simulink model "MIAC_Gain_or_disturbance_adaptive_test"  (R2018b)
settings: Solver=FixedStepDiscrete  StartTime=0.0  StopTime=60000  FixedStep=1  RelTol=1e-3
libraries: simulink x5, slident x5, powerlib_meascontrol x4
(part 2 of 3)

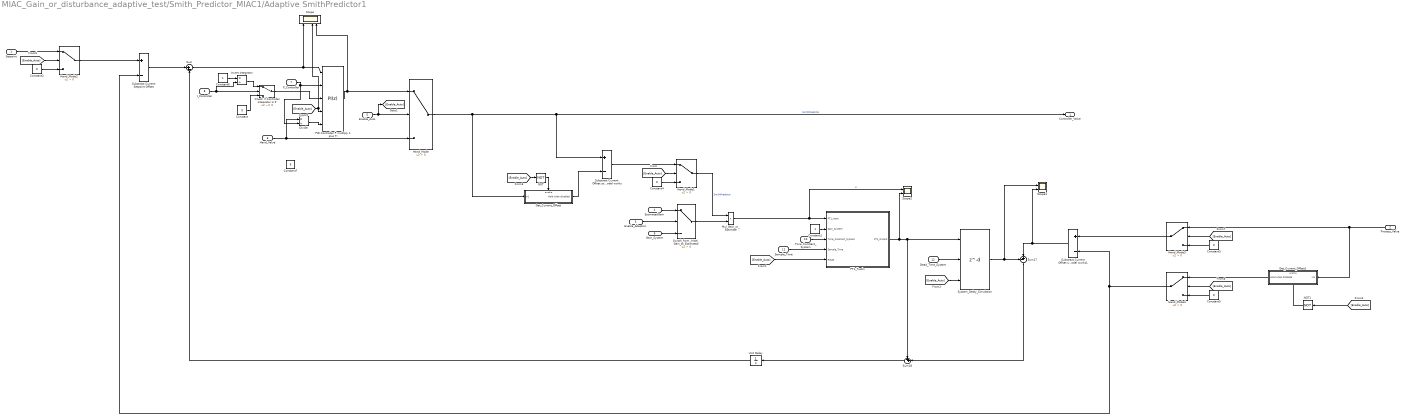
== system MIAC_Gain_or_disturbance_adaptive_test/Smith_Predictor_MIAC1/Adaptive SmithPredictor1 ==
  Setpoint : Inport
  Process_Value : Inport  Port=2
  Enable_Adaption : Inport  Port=3
  EstimatedGain : Inport  Port=4
  Enable_Auto : Inport  Port=5
  Hand_Value : Inport  Port=6
  P_Controller : Inport  Port=7
  I_Controller : Inport  Port=8
  Gain_System : Inport  Port=9
  Time_Constant_System : Inport  Port=10
  Sample_Time : Inport  Port=11
  " Dead_Time_System" : Inport  Port=12
  Check if Controller Integrator is 0 : Switch  Criteria=u2 ~= 0
  Constant{,2..5} (5 alike) : Constant  Value=0
  Constant1 : Constant
  Constant6 : Constant
  Constant7 : Constant  Value=6
  Divide : Product  Inputs=*/
  Get_Current_Offset : Subsystem
  Get_Current_Offset1 : Subsystem
  Hand_Mode{,1..4} (5 alike) : Switch  Criteria=u2 > Threshold
  Invert Integrator : Product  Inputs=*/
  Mul_Gain_or_Estimate : Product
  NOT : Logic  Operator=NOT  IconShape=distinctive  AllPortsSameDT=off  OutDataTypeStr=boolean
  NOT1 : Logic  Operator=NOT  IconShape=distinctive  AllPortsSameDT=off  OutDataTypeStr=boolean
  "PID Controller P multiply 1 plus Ti " : simulink/Continuous/PID Controller  Controller=PI  Form=Ideal  TimeDomain=Discrete-time  SampleTime=1  IntegratorMethod=Forward Euler  FilterMethod=Forward Euler  ControllerParametersSource=external  P=1.66148812255363  I=0.0833845225035065  D=118.272348286844  UseFilter=on  N=0.00420306193364532  TunerSelectOption=Transfer Function Based (PID Tuner App)  InitialConditionSource=external  InitialConditionForIntegrator=0  InitialConditionForFilter=0  DifferentiatorICPrevScaledInput=0  ExternalReset=rising  TrackingMode=off  Kt=1  LimitOutput=on  UpperSaturationLimit=100  LowerSaturationLimit=0  LinearizeAsGain=on  AntiWindupMode=none  Kb=1  POutMin=[]  POutMax=[]  IOutMin=[]  IOutMax=[]  DOutMin=[]  DOutMax=[]  NOutMin=[]  NOutMax=[]  SumOutMin=[]  SumOutMax=[]  SaturationOutMin=[]  SaturationOutMax=[]  PParamMin=[]  PParamMax=[]  IParamMin=[]  IParamMax=[]  DParamMin=[]  DParamMax=[]  NParamMin=[]  NParamMax=[]  KbParamMin=[]  KbParamMax=[]  KtParamMin=[]  KtParamMax=[]  KbOutMin=[]  KbOutMax=[]  KtOutMin=[]  KtOutMax=[]  IntegratorOutMin=[]  IntegratorOutMax=[]  FilterOutMin=[]  FilterOutMax=[]  SumI1OutMin=[]  SumI1OutMax=[]  SumI2OutMin=[]  SumI2OutMax=[]  SumI3OutMin=[]  SumI3OutMax=[]  SumI4OutMin=[]  SumI4OutMax=[]  SumDOutMin=[]  SumDOutMax=[]  DifferentiatorOutMin=[]  DifferentiatorOutMax=[]  FilterDiffOutCoefMin=[]  FilterDiffOutCoefMax=[]  ReciprocalOutMin=[]  ReciprocalOutMax=[]  SumDenOutMin=[]  SumDenOutMax=[]  SumNumOutMin=[]  SumNumOutMax=[]  DivideOutMin=[]  DivideOutMax=[]  IntegratorContinuousStateAttributes=''  IntegratorStateMustResolveToSignalObject=off  IntegratorRTWStateStorageClass=Auto  FilterContinuousStateAttributes=''  FilterStateMustResolveToSignalObject=off  FilterRTWStateStorageClass=Auto  ParallelPVariant=Passthrough  IdealPVariant=ExternalParameters  IVariant=ExternalParameters  DVariant=Disabled  IntegratorVariant=Discrete  SatVariant=Enabled  AWVariant=Passthrough  PCopyVariant=Disabled  TRVariant=Disabled  FdbkBlocksVariant=Forward  IdealPFdbkVariant=Disabled  SatFdbkVariant=Disabled  DerivativeFilterVariant=Disabled  NVariant=Disabled  NCopyVariant=Disabled_SignalSpec  FilterICVariant=Disabled  IntegratorICVariant=ExternalICs  ExternalResetVariant=ExternalReset  TRSumVariant=Passthrough  SumFdbkVariant=Disabled  SumVariant=Sum_PI
  PT1_Tustin : Subsystem  TreatAsAtomicUnit=on  SystemSampleTime=1
  Scope : Scope  NumInputPorts=4
  Scope1 : Scope  NumInputPorts=2
  Scope2 : Scope  NumInputPorts=2
  Substract Current Offset so that the linearised model works : Sum  Inputs=+-
  Substract Current Offset so that the linearised model works1 : Sum  Inputs=+-
  Substract Current Setpoint Offset : Sum  Inputs=+-
  Sum : Sum  Inputs=|+-
  Sum17 : Sum  Inputs=-+|
  Sum18 : Sum  Inputs=++|
  Switch_from_initial_Gain_to_Estimated : Switch  Criteria=u2 > Threshold
  System_Delay_Simulation : Delay  DelayLengthSource=Input port  DelayLength=600  DelayLengthUpperLimit=800  ExternalReset=Rising  SampleTime=1
      settings: InputPortMap=u0,p1,r5
  Unit Delay : UnitDelay
  Controller_Value : Outport
  wires:
  Substract Current Setpoint Offset/1 -> Sum/1
  Sum/1 -> "PID Controller P multiply 1 plus Ti "/1, Scope/1
  Hand_Mode/1 -> Get_Current_Offset/1(In1), Controller_Value/1, Substract Current Offset so that the linearised model works/1  "SmithPredictor"
  Substract Current Offset so that the linearised model works1/1 -> Scope1/2, Sum17/2
  PT1_Tustin/1(PT1_Output) -> Scope2/2, Sum18/1, System_Delay_Simulation/1
  System_Delay_Simulation/1 -> Scope1/1, Sum17/1
  Sum17/1 -> Sum18/2
  Mul_Gain_or_Estimate/1 -> Scope2/1, PT1_Tustin/1(PT1_Input)  "U"
  Switch_from_initial_Gain_to_Estimated/1 -> Mul_Gain_or_Estimate/2
  "PID Controller P multiply 1 plus Ti "/1 -> Hand_Mode/1, Scope/4
  Hand_Value/1 -> Divide/1, Hand_Mode/3
  Enable_Auto/1 -> [Enable_Auto], Hand_Mode/2
  P_Controller/1 -> "PID Controller P multiply 1 plus Ti "/2, Divide/2
  Check if Controller Integrator is 0/1 -> "PID Controller P multiply 1 plus Ti "/3
  " Dead_Time_System"/1 -> System_Delay_Simulation/2
  Gain_System/1 -> Switch_from_initial_Gain_to_Estimated/3
  Enable_Adaption/1 -> Switch_from_initial_Gain_to_Estimated/2
  EstimatedGain/1 -> Switch_from_initial_Gain_to_Estimated/1
  [Enable_Auto] -> Hand_Mode1/2
  Hand_Mode1/1 -> Mul_Gain_or_Estimate/1  "SmithPredictor"
  Constant4/1 -> Hand_Mode1/3
  [Enable_Auto] -> PT1_Tustin/5(Reset)
  [Enable_Auto] -> System_Delay_Simulation/3
  Substract Current Offset so that the linearised model works/1 -> Hand_Mode1/1
  Get_Current_Offset/1(Hold when disabled) -> Substract Current Offset so that the linearised model works/2
  [Enable_Auto] -> NOT/1
  NOT/1 -> Get_Current_Offset/Enable
  Sum18/1 -> Unit Delay/1
  Hand_Mode2/1 -> Substract Current Setpoint Offset/1
  NOT1/1 -> Get_Current_Offset1/Enable
  [Enable_Auto] -> NOT1/1
  Hand_Mode4/1 -> Substract Current Setpoint Offset/2, Substract Current Offset so that the linearised model works1/2
  Setpoint/1 -> Hand_Mode2/1
  [Enable_Auto] -> Hand_Mode2/2
  Constant2/1 -> Hand_Mode2/3
  Process_Value/1 -> Get_Current_Offset1/1(In1), Hand_Mode3/1
  [Enable_Auto] -> Hand_Mode3/2
  Constant3/1 -> Hand_Mode3/3
  Hand_Mode3/1 -> Substract Current Offset so that the linearised model works1/1
  Constant5/1 -> Hand_Mode4/3
  [Enable_Auto] -> Hand_Mode4/2
  Get_Current_Offset1/1(Hold when disabled) -> Hand_Mode4/1
  Time_Constant_System/1 -> PT1_Tustin/3(Time_Constant_System)
  Constant1/1 -> PT1_Tustin/2(Gain_System)
  Sample_Time/1 -> PT1_Tustin/4(Sample_Time)
  I_Controller/1 -> Check if Controller Integrator is 0/2, Invert Integrator/2
  Constant/1 -> Check if Controller Integrator is 0/3
  Invert Integrator/1 -> Check if Controller Integrator is 0/1
  Constant6/1 -> Invert Integrator/1
  Unit Delay/1 -> Sum/2
  [Enable_Auto] -> Scope/3, "PID Controller P multiply 1 plus Ti "/4
  Divide/1 -> "PID Controller P multiply 1 plus Ti "/5

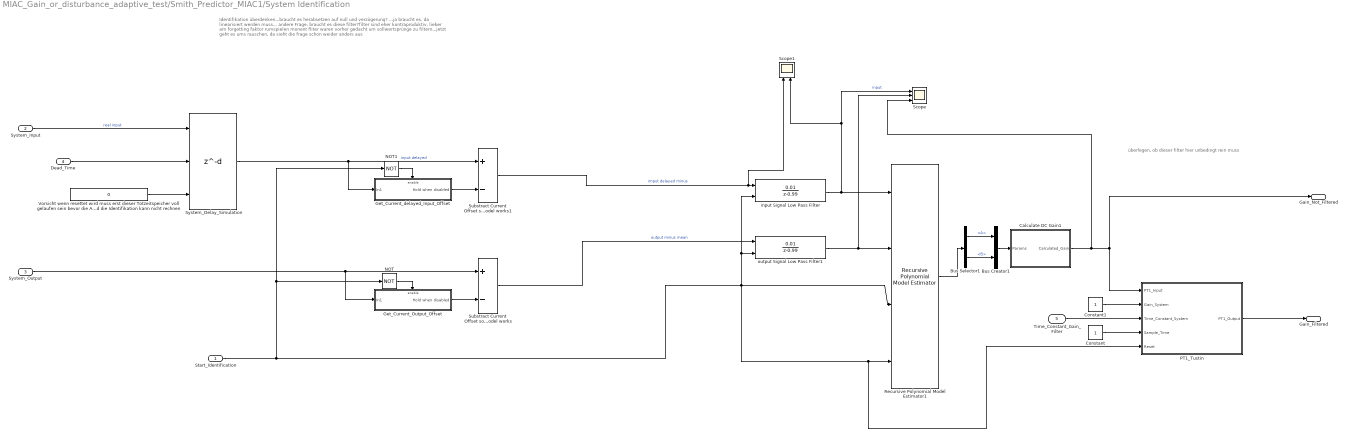
== system MIAC_Gain_or_disturbance_adaptive_test/Smith_Predictor_MIAC1/System Identification ==
  note: überlegen, ob dieser filter hier unbedingt rein muss
  note: Identifikation überdenken...braucht es herabsetzen auf null und verzögerung?
      | ...ja braucht es, da linearisiert werden muss...
      |
      | andere Frage, braucht es diese filter?filter sind eher kontraproduktiv, lieber am forgetting faktor rumspielen
      | monent fliter waren vorher gedacht um sollwertsprünge zu filtern...jetzt geht es ums rauschen, da sieht die frage schon weider anders aus
  Start_Identification : Inport  SampleTime=1
  System_Input : Inport  Port=2
  System_Output : Inport  Port=3  SampleTime=1
  Dead_Time : Inport  Port=4
  Time_Constant_Gain_Filter : Inport  Port=5
  Bus Creator1 : BusCreator  Inputs=2
  Bus Selector1 : BusSelector  OutputSignals=A,B
  Calculate DC Gain1 : Subsystem  TreatAsAtomicUnit=on  SystemSampleTime=1
  Constant : Constant
  Constant1 : Constant
  Get_Current_Output_Offset : Subsystem
  Get_Current_delayed_Input_Offset : Subsystem
  NOT : Logic  Operator=NOT  IconShape=distinctive  AllPortsSameDT=off  OutDataTypeStr=boolean
  NOT1 : Logic  Operator=NOT  IconShape=distinctive  AllPortsSameDT=off  OutDataTypeStr=boolean
  PT1_Tustin : Subsystem  TreatAsAtomicUnit=on  SystemSampleTime=1
  Recursive Polynomial Model Estimator1 : slident/Estimators/Recursive Polynomial Model Estimator  ModelStructure=ARX  InitialEstimateSource=None  A0=2  B0=1  C0=1  D0=1  F0=1  nk=1  P0=10  InitialInputs=0  InitialOutputs=0  History=Infinite  WindowLength=2000  EstimationMethod=Forgetting Factor  AdaptationParameter=1  HasTimeVaryingAdaptationParameter=off  NormalizationBias=eps  OutputError=off  OutputP=off  AddEnablePort=on  ExternalReset=Rising  InputProcessing=Sample-based  Ts=1
      settings: SourceProductName=System Identification Toolbox  SourceProductBaseCode=ID
  Scope : Scope  NumInputPorts=3
  Scope1 : Scope  NumInputPorts=2
  Substract Current Offset so that the linearised model works : Sum  Inputs=+-
  Substract Current Offset so that the linearised model works1 : Sum  Inputs=+-
  System_Delay_Simulation : Delay  DelayLengthSource=Input port  DelayLength=600  DelayLengthUpperLimit=800  ExternalReset=Rising  SampleTime=1
      settings: InputPortMap=u0,p1,r5
  Vorsicht wenn resettet wird muss erst dieser Totzeitspeicher voll gelaufen sein bevor die Adaption starten darf Sonst kommt heir immer 0 raus und die Identifikation kann nicht rechnen : Constant  Value=0
  input Signal Low Pass Filter : DiscreteTransferFcn  Numerator=[0.01]  Denominator=[1 -0.99]  ExternalReset=Rising  SampleTime=1  a0EqualsOne=on
      settings: InputPortMap=u0,r7
  output Signal Low Pass Filter1 : DiscreteTransferFcn  Numerator=[0.01]  Denominator=[1 -0.99]  ExternalReset=Rising  SampleTime=1  a0EqualsOne=on
      settings: InputPortMap=u0,r7
  Gain_Filtered : Outport
  Gain_Not_Filtered : Outport  Port=2
  wires:
  Recursive Polynomial Model Estimator1/1 -> Bus Selector1/1
  input Signal Low Pass Filter/1 -> Scope1/2, Scope/1, Recursive Polynomial Model Estimator1/1  "input"
  Bus Creator1/1 -> Calculate DC Gain1/1(Params)
  Bus Selector1/1 -> Bus Creator1/1  "<A>"
  Bus Selector1/2 -> Bus Creator1/2  "<B>"
  Substract Current Offset so that the linearised model works/1 -> output Signal Low Pass Filter1/1  "output minus mean"
  NOT/1 -> Get_Current_Output_Offset/Enable
  Get_Current_Output_Offset/1(Hold when disabled) -> Substract Current Offset so that the linearised model works/2
  System_Output/1 -> Get_Current_Output_Offset/1(In1), Substract Current Offset so that the linearised model works/1
  Get_Current_delayed_Input_Offset/1(Hold when disabled) -> Substract Current Offset so that the linearised model works1/2
  NOT1/1 -> Get_Current_delayed_Input_Offset/Enable
  PT1_Tustin/1(PT1_Output) -> Gain_Filtered/1
  System_Input/1 -> System_Delay_Simulation/1  "real input"
  Vorsicht wenn resettet wird muss erst dieser Totzeitspeicher voll gelaufen sein bevor die Adaption starten darf Sonst kommt heir immer 0 raus und die Identifikation kann nicht rechnen/1 -> System_Delay_Simulation/3
  Dead_Time/1 -> System_Delay_Simulation/2
  Substract Current Offset so that the linearised model works1/1 -> Scope1/1, input Signal Low Pass Filter/1  "imput delayed minus"
  System_Delay_Simulation/1 -> Substract Current Offset so that the linearised model works1/1, Get_Current_delayed_Input_Offset/1(In1)  "input delayed"
  Calculate DC Gain1/1(Calculated_Gain) -> Scope/3, PT1_Tustin/1(PT1_Input), Gain_Not_Filtered/1
  Start_Identification/1 -> NOT/1, NOT1/1, PT1_Tustin/5(Reset), Recursive Polynomial Model Estimator1/4, output Signal Low Pass Filter1/2, input Signal Low Pass Filter/2, Recursive Polynomial Model Estimator1/3
  output Signal Low Pass Filter1/1 -> Scope/2, Recursive Polynomial Model Estimator1/2
  Constant/1 -> PT1_Tustin/4(Sample_Time)
  Constant1/1 -> PT1_Tustin/2(Gain_System)
  Time_Constant_Gain_Filter/1 -> PT1_Tustin/3(Time_Constant_System)

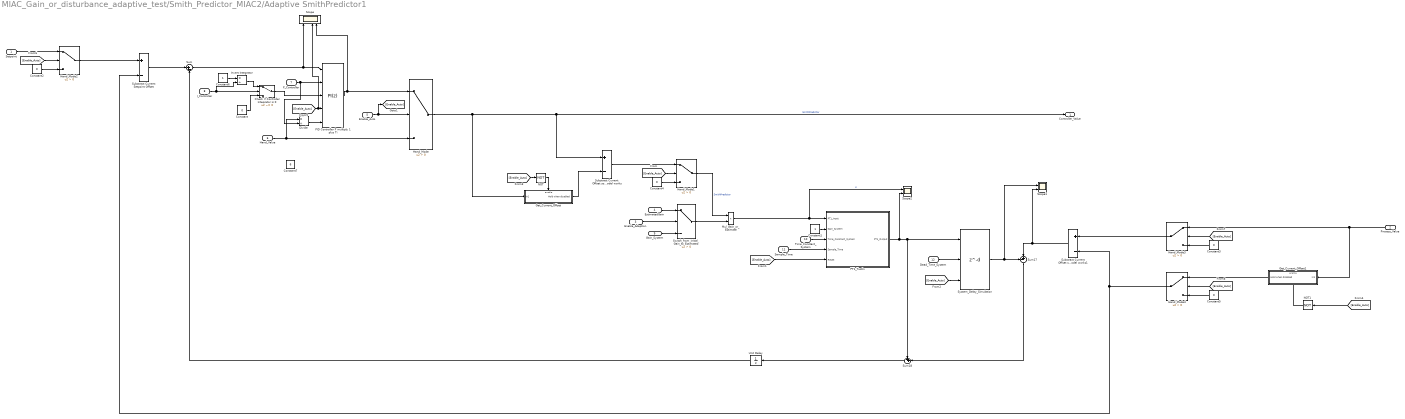
== system MIAC_Gain_or_disturbance_adaptive_test/Smith_Predictor_MIAC2/Adaptive SmithPredictor1 ==
  Setpoint : Inport
  Process_Value : Inport  Port=2
  Enable_Adaption : Inport  Port=3
  EstimatedGain : Inport  Port=4
  Enable_Auto : Inport  Port=5
  Hand_Value : Inport  Port=6
  P_Controller : Inport  Port=7
  I_Controller : Inport  Port=8
  Gain_System : Inport  Port=9
  Time_Constant_System : Inport  Port=10
  Sample_Time : Inport  Port=11
  " Dead_Time_System" : Inport  Port=12
  Check if Controller Integrator is 0 : Switch  Criteria=u2 ~= 0
  Constant{,2..5} (5 alike) : Constant  Value=0
  Constant1 : Constant
  Constant6 : Constant
  Constant7 : Constant  Value=6
  Divide : Product  Inputs=*/
  Get_Current_Offset : Subsystem
  Get_Current_Offset1 : Subsystem
  Hand_Mode{,1..4} (5 alike) : Switch  Criteria=u2 > Threshold
  Invert Integrator : Product  Inputs=*/
  Mul_Gain_or_Estimate : Product
  NOT : Logic  Operator=NOT  IconShape=distinctive  AllPortsSameDT=off  OutDataTypeStr=boolean
  NOT1 : Logic  Operator=NOT  IconShape=distinctive  AllPortsSameDT=off  OutDataTypeStr=boolean
  "PID Controller P multiply 1 plus Ti " : simulink/Continuous/PID Controller  Controller=PI  Form=Ideal  TimeDomain=Discrete-time  SampleTime=1  IntegratorMethod=Forward Euler  FilterMethod=Forward Euler  ControllerParametersSource=external  P=3.04732259067536  I=0.00445689106465138  D=118.272348286844  UseFilter=on  N=0.00420306193364532  TunerSelectOption=Transfer Function Based (PID Tuner App)  InitialConditionSource=external  InitialConditionForIntegrator=0  InitialConditionForFilter=0  DifferentiatorICPrevScaledInput=0  ExternalReset=rising  TrackingMode=off  Kt=1  LimitOutput=on  UpperSaturationLimit=100  LowerSaturationLimit=0  LinearizeAsGain=on  AntiWindupMode=none  Kb=1  POutMin=[]  POutMax=[]  IOutMin=[]  IOutMax=[]  DOutMin=[]  DOutMax=[]  NOutMin=[]  NOutMax=[]  SumOutMin=[]  SumOutMax=[]  SaturationOutMin=[]  SaturationOutMax=[]  PParamMin=[]  PParamMax=[]  IParamMin=[]  IParamMax=[]  DParamMin=[]  DParamMax=[]  NParamMin=[]  NParamMax=[]  KbParamMin=[]  KbParamMax=[]  KtParamMin=[]  KtParamMax=[]  KbOutMin=[]  KbOutMax=[]  KtOutMin=[]  KtOutMax=[]  IntegratorOutMin=[]  IntegratorOutMax=[]  FilterOutMin=[]  FilterOutMax=[]  SumI1OutMin=[]  SumI1OutMax=[]  SumI2OutMin=[]  SumI2OutMax=[]  SumI3OutMin=[]  SumI3OutMax=[]  SumI4OutMin=[]  SumI4OutMax=[]  SumDOutMin=[]  SumDOutMax=[]  DifferentiatorOutMin=[]  DifferentiatorOutMax=[]  FilterDiffOutCoefMin=[]  FilterDiffOutCoefMax=[]  ReciprocalOutMin=[]  ReciprocalOutMax=[]  SumDenOutMin=[]  SumDenOutMax=[]  SumNumOutMin=[]  SumNumOutMax=[]  DivideOutMin=[]  DivideOutMax=[]  IntegratorContinuousStateAttributes=''  IntegratorStateMustResolveToSignalObject=off  IntegratorRTWStateStorageClass=Auto  FilterContinuousStateAttributes=''  FilterStateMustResolveToSignalObject=off  FilterRTWStateStorageClass=Auto  ParallelPVariant=Passthrough  IdealPVariant=ExternalParameters  IVariant=ExternalParameters  DVariant=Disabled  IntegratorVariant=Discrete  SatVariant=Enabled  AWVariant=Passthrough  PCopyVariant=Disabled  TRVariant=Disabled  FdbkBlocksVariant=Forward  IdealPFdbkVariant=Disabled  SatFdbkVariant=Disabled  DerivativeFilterVariant=Disabled  NVariant=Disabled  NCopyVariant=Disabled_SignalSpec  FilterICVariant=Disabled  IntegratorICVariant=ExternalICs  ExternalResetVariant=ExternalReset  TRSumVariant=Passthrough  SumFdbkVariant=Disabled  SumVariant=Sum_PI
  PT1_Tustin : Subsystem  TreatAsAtomicUnit=on  SystemSampleTime=1
  Scope : Scope  NumInputPorts=4
  Scope1 : Scope  NumInputPorts=2
  Scope2 : Scope  NumInputPorts=2
  Substract Current Offset so that the linearised model works : Sum  Inputs=+-
  Substract Current Offset so that the linearised model works1 : Sum  Inputs=+-
  Substract Current Setpoint Offset : Sum  Inputs=+-
  Sum : Sum  Inputs=|+-
  Sum17 : Sum  Inputs=-+|
  Sum18 : Sum  Inputs=++|
  Switch_from_initial_Gain_to_Estimated : Switch  Criteria=u2 > Threshold
  System_Delay_Simulation : Delay  DelayLengthSource=Input port  DelayLength=600  DelayLengthUpperLimit=800  ExternalReset=Rising  SampleTime=1
      settings: InputPortMap=u0,p1,r5
  Unit Delay : UnitDelay
  Controller_Value : Outport
  wires:
  Substract Current Setpoint Offset/1 -> Sum/1
  Sum/1 -> "PID Controller P multiply 1 plus Ti "/1, Scope/1
  Hand_Mode/1 -> Get_Current_Offset/1(In1), Controller_Value/1, Substract Current Offset so that the linearised model works/1  "SmithPredictor"
  Substract Current Offset so that the linearised model works1/1 -> Scope1/2, Sum17/2
  PT1_Tustin/1(PT1_Output) -> Scope2/2, Sum18/1, System_Delay_Simulation/1
  System_Delay_Simulation/1 -> Scope1/1, Sum17/1
  Sum17/1 -> Sum18/2
  Mul_Gain_or_Estimate/1 -> Scope2/1, PT1_Tustin/1(PT1_Input)  "U"
  Switch_from_initial_Gain_to_Estimated/1 -> Mul_Gain_or_Estimate/2
  "PID Controller P multiply 1 plus Ti "/1 -> Hand_Mode/1, Scope/4
  Hand_Value/1 -> Divide/1, Hand_Mode/3
  Enable_Auto/1 -> [Enable_Auto], Hand_Mode/2
  P_Controller/1 -> Divide/2, "PID Controller P multiply 1 plus Ti "/2
  Check if Controller Integrator is 0/1 -> "PID Controller P multiply 1 plus Ti "/3
  " Dead_Time_System"/1 -> System_Delay_Simulation/2
  Gain_System/1 -> Switch_from_initial_Gain_to_Estimated/3
  Enable_Adaption/1 -> Switch_from_initial_Gain_to_Estimated/2
  EstimatedGain/1 -> Switch_from_initial_Gain_to_Estimated/1
  [Enable_Auto] -> Hand_Mode1/2
  Hand_Mode1/1 -> Mul_Gain_or_Estimate/1  "SmithPredictor"
  Constant4/1 -> Hand_Mode1/3
  [Enable_Auto] -> PT1_Tustin/5(Reset)
  [Enable_Auto] -> System_Delay_Simulation/3
  Substract Current Offset so that the linearised model works/1 -> Hand_Mode1/1
  Get_Current_Offset/1(Hold when disabled) -> Substract Current Offset so that the linearised model works/2
  [Enable_Auto] -> NOT/1
  NOT/1 -> Get_Current_Offset/Enable
  Sum18/1 -> Unit Delay/1
  Hand_Mode2/1 -> Substract Current Setpoint Offset/1
  NOT1/1 -> Get_Current_Offset1/Enable
  [Enable_Auto] -> NOT1/1
  Hand_Mode4/1 -> Substract Current Setpoint Offset/2, Substract Current Offset so that the linearised model works1/2
  Setpoint/1 -> Hand_Mode2/1
  [Enable_Auto] -> Hand_Mode2/2
  Constant2/1 -> Hand_Mode2/3
  Process_Value/1 -> Get_Current_Offset1/1(In1), Hand_Mode3/1
  [Enable_Auto] -> Hand_Mode3/2
  Constant3/1 -> Hand_Mode3/3
  Hand_Mode3/1 -> Substract Current Offset so that the linearised model works1/1
  Constant5/1 -> Hand_Mode4/3
  [Enable_Auto] -> Hand_Mode4/2
  Get_Current_Offset1/1(Hold when disabled) -> Hand_Mode4/1
  Time_Constant_System/1 -> PT1_Tustin/3(Time_Constant_System)
  Constant1/1 -> PT1_Tustin/2(Gain_System)
  Sample_Time/1 -> PT1_Tustin/4(Sample_Time)
  I_Controller/1 -> Check if Controller Integrator is 0/2, Invert Integrator/2
  Constant/1 -> Check if Controller Integrator is 0/3
  Invert Integrator/1 -> Check if Controller Integrator is 0/1
  Constant6/1 -> Invert Integrator/1
  Unit Delay/1 -> Sum/2
  [Enable_Auto] -> Scope/3, "PID Controller P multiply 1 plus Ti "/4
  Divide/1 -> "PID Controller P multiply 1 plus Ti "/5

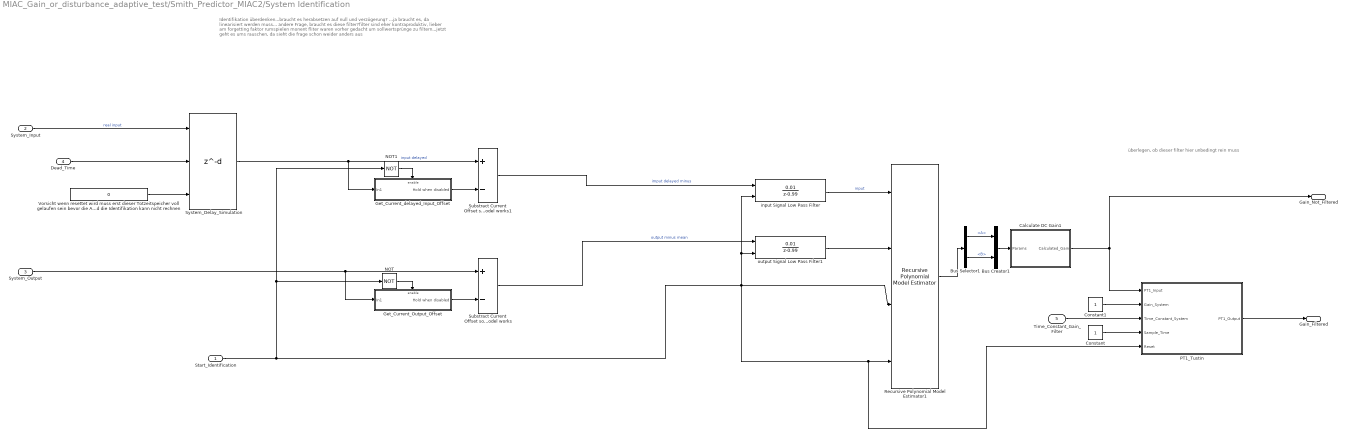
== system MIAC_Gain_or_disturbance_adaptive_test/Smith_Predictor_MIAC2/System Identification ==
  note: überlegen, ob dieser filter hier unbedingt rein muss
  note: Identifikation überdenken...braucht es herabsetzen auf null und verzögerung?
      | ...ja braucht es, da linearisiert werden muss...
      |
      | andere Frage, braucht es diese filter?filter sind eher kontraproduktiv, lieber am forgetting faktor rumspielen
      | monent fliter waren vorher gedacht um sollwertsprünge zu filtern...jetzt geht es ums rauschen, da sieht die frage schon weider anders aus
  Start_Identification : Inport  SampleTime=1
  System_Input : Inport  Port=2
  System_Output : Inport  Port=3  SampleTime=1
  Dead_Time : Inport  Port=4
  Time_Constant_Gain_Filter : Inport  Port=5
  Bus Creator1 : BusCreator  Inputs=2
  Bus Selector1 : BusSelector  OutputSignals=A,B
  Calculate DC Gain1 : Subsystem  TreatAsAtomicUnit=on  SystemSampleTime=1
  Constant : Constant
  Constant1 : Constant
  Get_Current_Output_Offset : Subsystem
  Get_Current_delayed_Input_Offset : Subsystem
  NOT : Logic  Operator=NOT  IconShape=distinctive  AllPortsSameDT=off  OutDataTypeStr=boolean
  NOT1 : Logic  Operator=NOT  IconShape=distinctive  AllPortsSameDT=off  OutDataTypeStr=boolean
  PT1_Tustin : Subsystem  TreatAsAtomicUnit=on  SystemSampleTime=1
  Recursive Polynomial Model Estimator1 : slident/Estimators/Recursive Polynomial Model Estimator  ModelStructure=ARX  InitialEstimateSource=None  A0=2  B0=1  C0=1  D0=1  F0=1  nk=1  P0=10  InitialInputs=0  InitialOutputs=0  History=Infinite  WindowLength=2000  EstimationMethod=Forgetting Factor  AdaptationParameter=1  HasTimeVaryingAdaptationParameter=off  NormalizationBias=eps  OutputError=off  OutputP=off  AddEnablePort=on  ExternalReset=Rising  InputProcessing=Sample-based  Ts=1
      settings: SourceProductName=System Identification Toolbox  SourceProductBaseCode=ID
  Substract Current Offset so that the linearised model works : Sum  Inputs=+-
  Substract Current Offset so that the linearised model works1 : Sum  Inputs=+-
  System_Delay_Simulation : Delay  DelayLengthSource=Input port  DelayLength=600  DelayLengthUpperLimit=800  ExternalReset=Rising  SampleTime=1
      settings: InputPortMap=u0,p1,r5
  Vorsicht wenn resettet wird muss erst dieser Totzeitspeicher voll gelaufen sein bevor die Adaption starten darf Sonst kommt heir immer 0 raus und die Identifikation kann nicht rechnen : Constant  Value=0
  input Signal Low Pass Filter : DiscreteTransferFcn  Numerator=[0.01]  Denominator=[1 -0.99]  ExternalReset=Rising  SampleTime=1  a0EqualsOne=on
      settings: InputPortMap=u0,r7
  output Signal Low Pass Filter1 : DiscreteTransferFcn  Numerator=[0.01]  Denominator=[1 -0.99]  ExternalReset=Rising  SampleTime=1  a0EqualsOne=on
      settings: InputPortMap=u0,r7
  Gain_Filtered : Outport
  Gain_Not_Filtered : Outport  Port=2
  wires:
  Recursive Polynomial Model Estimator1/1 -> Bus Selector1/1
  input Signal Low Pass Filter/1 -> Recursive Polynomial Model Estimator1/1  "input"
  Bus Creator1/1 -> Calculate DC Gain1/1(Params)
  Bus Selector1/1 -> Bus Creator1/1  "<A>"
  Bus Selector1/2 -> Bus Creator1/2  "<B>"
  Substract Current Offset so that the linearised model works/1 -> output Signal Low Pass Filter1/1  "output minus mean"
  NOT/1 -> Get_Current_Output_Offset/Enable
  Get_Current_Output_Offset/1(Hold when disabled) -> Substract Current Offset so that the linearised model works/2
  System_Output/1 -> Get_Current_Output_Offset/1(In1), Substract Current Offset so that the linearised model works/1
  Get_Current_delayed_Input_Offset/1(Hold when disabled) -> Substract Current Offset so that the linearised model works1/2
  NOT1/1 -> Get_Current_delayed_Input_Offset/Enable
  PT1_Tustin/1(PT1_Output) -> Gain_Filtered/1
  System_Input/1 -> System_Delay_Simulation/1  "real input"
  Vorsicht wenn resettet wird muss erst dieser Totzeitspeicher voll gelaufen sein bevor die Adaption starten darf Sonst kommt heir immer 0 raus und die Identifikation kann nicht rechnen/1 -> System_Delay_Simulation/3
  Dead_Time/1 -> System_Delay_Simulation/2
  Substract Current Offset so that the linearised model works1/1 -> input Signal Low Pass Filter/1  "imput delayed minus"
  System_Delay_Simulation/1 -> Substract Current Offset so that the linearised model works1/1, Get_Current_delayed_Input_Offset/1(In1)  "input delayed"
  Calculate DC Gain1/1(Calculated_Gain) -> PT1_Tustin/1(PT1_Input), Gain_Not_Filtered/1
  Start_Identification/1 -> NOT/1, NOT1/1, PT1_Tustin/5(Reset), Recursive Polynomial Model Estimator1/4, output Signal Low Pass Filter1/2, input Signal Low Pass Filter/2, Recursive Polynomial Model Estimator1/3
  output Signal Low Pass Filter1/1 -> Recursive Polynomial Model Estimator1/2
  Constant/1 -> PT1_Tustin/4(Sample_Time)
  Constant1/1 -> PT1_Tustin/2(Gain_System)
  Time_Constant_Gain_Filter/1 -> PT1_Tustin/3(Time_Constant_System)

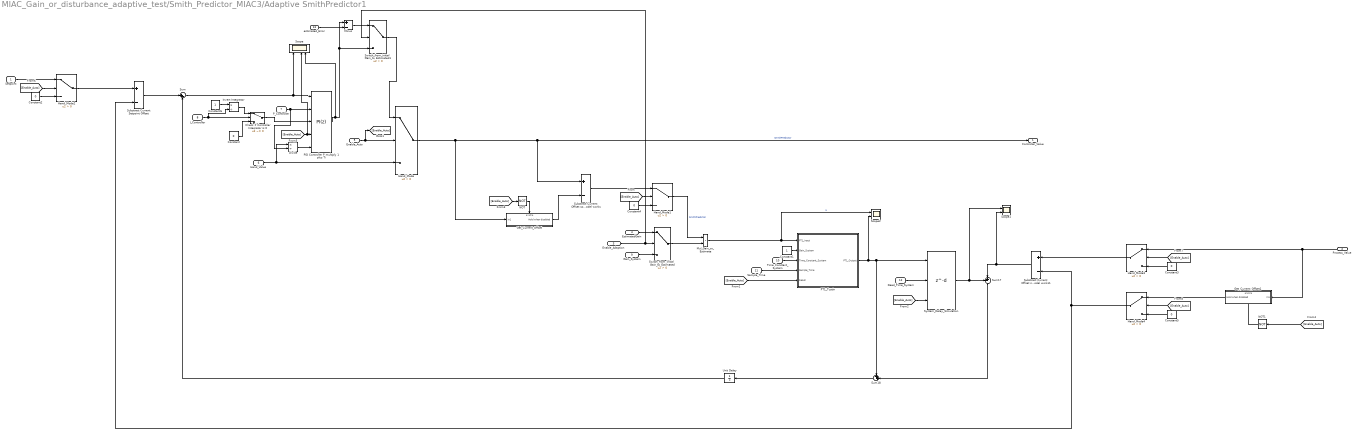
== system MIAC_Gain_or_disturbance_adaptive_test/Smith_Predictor_MIAC3/Adaptive SmithPredictor1 ==
  Setpoint : Inport
  Process_Value : Inport  Port=2
  Enable_Adaption : Inport  Port=3
  EstimatedGain : Inport  Port=4
  Enable_Auto : Inport  Port=5
  Hand_Value : Inport  Port=6
  P_Controller : Inport  Port=7
  I_Controller : Inport  Port=8
  Gain_System : Inport  Port=9
  Time_Constant_System : Inport  Port=10
  Sample_Time : Inport  Port=11
  " Dead_Time_System" : Inport  Port=12
  estimated_Error : Inport  Port=13
  Check if Controller Integrator is 0 : Switch  Criteria=u2 ~= 0
  Constant{,2..5} (5 alike) : Constant  Value=0
  Constant1 : Constant
  Constant6 : Constant
  Divide : Product  Inputs=*/
  Get_Current_Offset : Subsystem
  Get_Current_Offset1 : Subsystem
  Hand_Mode{,1..4} (5 alike) : Switch  Criteria=u2 > Threshold
  Invert Integrator : Product  Inputs=*/
  Minus : Sum  Inputs=+-
  Mul_Gain_or_Estimate : Product
  NOT : Logic  Operator=NOT  IconShape=distinctive  AllPortsSameDT=off  OutDataTypeStr=boolean
  NOT1 : Logic  Operator=NOT  IconShape=distinctive  AllPortsSameDT=off  OutDataTypeStr=boolean
  "PID Controller P multiply 1 plus Ti " : simulink/Continuous/PID Controller  Controller=PI  Form=Ideal  TimeDomain=Discrete-time  SampleTime=1  IntegratorMethod=Forward Euler  FilterMethod=Forward Euler  ControllerParametersSource=external  P=3.04732259067536  I=0.00445689106465138  D=118.272348286844  UseFilter=on  N=0.00420306193364532  TunerSelectOption=Transfer Function Based (PID Tuner App)  InitialConditionSource=external  InitialConditionForIntegrator=0  InitialConditionForFilter=0  DifferentiatorICPrevScaledInput=0  ExternalReset=rising  TrackingMode=off  Kt=1  LimitOutput=on  UpperSaturationLimit=100  LowerSaturationLimit=0  LinearizeAsGain=on  AntiWindupMode=none  Kb=1  POutMin=[]  POutMax=[]  IOutMin=[]  IOutMax=[]  DOutMin=[]  DOutMax=[]  NOutMin=[]  NOutMax=[]  SumOutMin=[]  SumOutMax=[]  SaturationOutMin=[]  SaturationOutMax=[]  PParamMin=[]  PParamMax=[]  IParamMin=[]  IParamMax=[]  DParamMin=[]  DParamMax=[]  NParamMin=[]  NParamMax=[]  KbParamMin=[]  KbParamMax=[]  KtParamMin=[]  KtParamMax=[]  KbOutMin=[]  KbOutMax=[]  KtOutMin=[]  KtOutMax=[]  IntegratorOutMin=[]  IntegratorOutMax=[]  FilterOutMin=[]  FilterOutMax=[]  SumI1OutMin=[]  SumI1OutMax=[]  SumI2OutMin=[]  SumI2OutMax=[]  SumI3OutMin=[]  SumI3OutMax=[]  SumI4OutMin=[]  SumI4OutMax=[]  SumDOutMin=[]  SumDOutMax=[]  DifferentiatorOutMin=[]  DifferentiatorOutMax=[]  FilterDiffOutCoefMin=[]  FilterDiffOutCoefMax=[]  ReciprocalOutMin=[]  ReciprocalOutMax=[]  SumDenOutMin=[]  SumDenOutMax=[]  SumNumOutMin=[]  SumNumOutMax=[]  DivideOutMin=[]  DivideOutMax=[]  IntegratorContinuousStateAttributes=''  IntegratorStateMustResolveToSignalObject=off  IntegratorRTWStateStorageClass=Auto  FilterContinuousStateAttributes=''  FilterStateMustResolveToSignalObject=off  FilterRTWStateStorageClass=Auto  ParallelPVariant=Passthrough  IdealPVariant=ExternalParameters  IVariant=ExternalParameters  DVariant=Disabled  IntegratorVariant=Discrete  SatVariant=Enabled  AWVariant=Passthrough  PCopyVariant=Disabled  TRVariant=Disabled  FdbkBlocksVariant=Forward  IdealPFdbkVariant=Disabled  SatFdbkVariant=Disabled  DerivativeFilterVariant=Disabled  NVariant=Disabled  NCopyVariant=Disabled_SignalSpec  FilterICVariant=Disabled  IntegratorICVariant=ExternalICs  ExternalResetVariant=ExternalReset  TRSumVariant=Passthrough  SumFdbkVariant=Disabled  SumVariant=Sum_PI
  PT1_Tustin : Subsystem  TreatAsAtomicUnit=on  SystemSampleTime=1
  Scope : Scope  NumInputPorts=4
  Scope1 : Scope  NumInputPorts=2
  Scope2 : Scope  NumInputPorts=2
  Substract Current Offset so that the linearised model works : Sum  Inputs=+-
  Substract Current Offset so that the linearised model works1 : Sum  Inputs=+-
  Substract Current Setpoint Offset : Sum  Inputs=+-
  Sum : Sum  Inputs=|+-
  Sum17 : Sum  Inputs=-+|
  Sum18 : Sum  Inputs=++|
  Switch_from_initial_Gain_to_Estimated : Switch  Criteria=u2 > Threshold
  Switch_from_initial_Gain_to_Estimated1 : Switch  Criteria=u2 > Threshold
  System_Delay_Simulation : Delay  DelayLengthSource=Input port  DelayLength=600  DelayLengthUpperLimit=800  ExternalReset=Rising  SampleTime=1
      settings: InputPortMap=u0,p1,r5
  Unit Delay : UnitDelay
  Controller_Value : Outport
  wires:
  Substract Current Setpoint Offset/1 -> Sum/1
  Sum/1 -> "PID Controller P multiply 1 plus Ti "/1, Scope/1
  Hand_Mode/1 -> Get_Current_Offset/1(In1), Controller_Value/1, Substract Current Offset so that the linearised model works/1  "SmithPredictor"
  Substract Current Offset so that the linearised model works1/1 -> Scope1/2, Sum17/2
  PT1_Tustin/1(PT1_Output) -> Scope2/2, Sum18/1, System_Delay_Simulation/1
  System_Delay_Simulation/1 -> Scope1/1, Sum17/1
  Sum17/1 -> Sum18/2
  Mul_Gain_or_Estimate/1 -> Scope2/1, PT1_Tustin/1(PT1_Input)  "U"
  Switch_from_initial_Gain_to_Estimated/1 -> Mul_Gain_or_Estimate/2
  "PID Controller P multiply 1 plus Ti "/1 -> Minus/1, Switch_from_initial_Gain_to_Estimated1/3, Scope/4
  Hand_Value/1 -> Divide/1, Hand_Mode/3
  Enable_Auto/1 -> [Enable_Auto], Hand_Mode/2
  P_Controller/1 -> Divide/2, "PID Controller P multiply 1 plus Ti "/2
  Check if Controller Integrator is 0/1 -> "PID Controller P multiply 1 plus Ti "/3
  " Dead_Time_System"/1 -> System_Delay_Simulation/2
  Gain_System/1 -> Switch_from_initial_Gain_to_Estimated/3
  Enable_Adaption/1 -> Switch_from_initial_Gain_to_Estimated1/2, Switch_from_initial_Gain_to_Estimated/2
  EstimatedGain/1 -> Switch_from_initial_Gain_to_Estimated/1
  [Enable_Auto] -> Hand_Mode1/2
  Hand_Mode1/1 -> Mul_Gain_or_Estimate/1  "SmithPredictor"
  Constant4/1 -> Hand_Mode1/3
  [Enable_Auto] -> PT1_Tustin/5(Reset)
  [Enable_Auto] -> System_Delay_Simulation/3
  Substract Current Offset so that the linearised model works/1 -> Hand_Mode1/1
  Get_Current_Offset/1(Hold when disabled) -> Substract Current Offset so that the linearised model works/2
  [Enable_Auto] -> NOT/1
  NOT/1 -> Get_Current_Offset/Enable
  Sum18/1 -> Unit Delay/1
  Hand_Mode2/1 -> Substract Current Setpoint Offset/1
  NOT1/1 -> Get_Current_Offset1/Enable
  [Enable_Auto] -> NOT1/1
  Hand_Mode4/1 -> Substract Current Setpoint Offset/2, Substract Current Offset so that the linearised model works1/2
  Setpoint/1 -> Hand_Mode2/1
  [Enable_Auto] -> Hand_Mode2/2
  Constant2/1 -> Hand_Mode2/3
  Process_Value/1 -> Get_Current_Offset1/1(In1), Hand_Mode3/1
  [Enable_Auto] -> Hand_Mode3/2
  Constant3/1 -> Hand_Mode3/3
  Hand_Mode3/1 -> Substract Current Offset so that the linearised model works1/1
  Constant5/1 -> Hand_Mode4/3
  [Enable_Auto] -> Hand_Mode4/2
  Get_Current_Offset1/1(Hold when disabled) -> Hand_Mode4/1
  Time_Constant_System/1 -> PT1_Tustin/3(Time_Constant_System)
  Constant1/1 -> PT1_Tustin/2(Gain_System)
  Sample_Time/1 -> PT1_Tustin/4(Sample_Time)
  I_Controller/1 -> Check if Controller Integrator is 0/2, Invert Integrator/2
  Constant/1 -> Check if Controller Integrator is 0/3
  Invert Integrator/1 -> Check if Controller Integrator is 0/1
  Constant6/1 -> Invert Integrator/1
  Unit Delay/1 -> Sum/2
  [Enable_Auto] -> Scope/3, "PID Controller P multiply 1 plus Ti "/4
  Divide/1 -> "PID Controller P multiply 1 plus Ti "/5
  Switch_from_initial_Gain_to_Estimated1/1 -> Hand_Mode/1
  Minus/1 -> Switch_from_initial_Gain_to_Estimated1/1
  estimated_Error/1 -> Minus/2

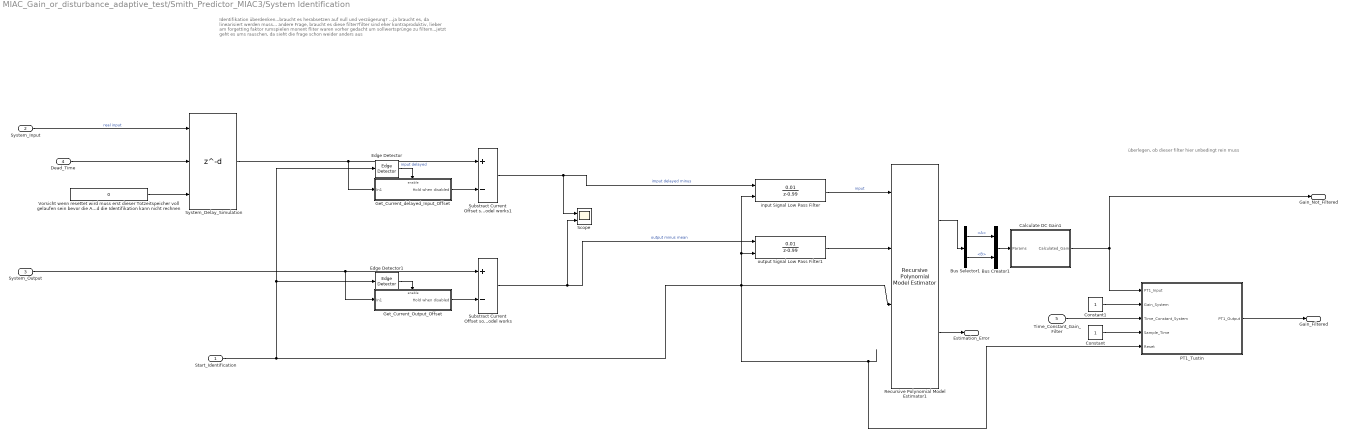
== system MIAC_Gain_or_disturbance_adaptive_test/Smith_Predictor_MIAC3/System Identification ==
  note: überlegen, ob dieser filter hier unbedingt rein muss
  note: Identifikation überdenken...braucht es herabsetzen auf null und verzögerung?
      | ...ja braucht es, da linearisiert werden muss...
      |
      | andere Frage, braucht es diese filter?filter sind eher kontraproduktiv, lieber am forgetting faktor rumspielen
      | monent fliter waren vorher gedacht um sollwertsprünge zu filtern...jetzt geht es ums rauschen, da sieht die frage schon weider anders aus
  Start_Identification : Inport  SampleTime=1
  System_Input : Inport  Port=2
  System_Output : Inport  Port=3  SampleTime=1
  Dead_Time : Inport  Port=4
  Time_Constant_Gain_Filter : Inport  Port=5
  Bus Creator1 : BusCreator  Inputs=2
  Bus Selector1 : BusSelector  OutputSignals=A,B
  Calculate DC Gain1 : Subsystem  TreatAsAtomicUnit=on  SystemSampleTime=1
  Constant : Constant
  Constant1 : Constant
  Edge Detector : powerlib_meascontrol/Logic/Edge Detector  model=Rising  ic=0  Ts=1
      settings: SourceProductName=Simscape Power Systems  SourceProductBaseCode=PS
  Edge Detector1 : powerlib_meascontrol/Logic/Edge Detector  model=Rising  ic=0  Ts=1
      settings: SourceProductName=Simscape Power Systems  SourceProductBaseCode=PS
  Get_Current_Output_Offset : Subsystem
  Get_Current_delayed_Input_Offset : Subsystem
  PT1_Tustin : Subsystem  TreatAsAtomicUnit=on  SystemSampleTime=1
  Recursive Polynomial Model Estimator1 : slident/Estimators/Recursive Polynomial Model Estimator  ModelStructure=ARX  InitialEstimateSource=None  A0=2  B0=1  C0=1  D0=1  F0=1  nk=1  P0=10  InitialInputs=0  InitialOutputs=0  History=Infinite  WindowLength=2000  EstimationMethod=Forgetting Factor  AdaptationParameter=1  HasTimeVaryingAdaptationParameter=off  NormalizationBias=eps  OutputError=on  OutputP=off  AddEnablePort=on  ExternalReset=Rising  InputProcessing=Sample-based  Ts=1
      settings: SourceProductName=System Identification Toolbox  SourceProductBaseCode=ID
  Scope : Scope  NumInputPorts=2
  Substract Current Offset so that the linearised model works : Sum  Inputs=+-
  Substract Current Offset so that the linearised model works1 : Sum  Inputs=+-
  System_Delay_Simulation : Delay  DelayLengthSource=Input port  DelayLength=600  DelayLengthUpperLimit=800  ExternalReset=Rising  SampleTime=1
      settings: InputPortMap=u0,p1,r5
  Vorsicht wenn resettet wird muss erst dieser Totzeitspeicher voll gelaufen sein bevor die Adaption starten darf Sonst kommt heir immer 0 raus und die Identifikation kann nicht rechnen : Constant  Value=0
  input Signal Low Pass Filter : DiscreteTransferFcn  Numerator=[0.01]  Denominator=[1 -0.99]  ExternalReset=Rising  SampleTime=1  a0EqualsOne=on
      settings: InputPortMap=u0,r7
  output Signal Low Pass Filter1 : DiscreteTransferFcn  Numerator=[0.01]  Denominator=[1 -0.99]  ExternalReset=Rising  SampleTime=1  a0EqualsOne=on
      settings: InputPortMap=u0,r7
  Gain_Filtered : Outport
  Gain_Not_Filtered : Outport  Port=2
  Estimation_Error : Outport  Port=3
  wires:
  Recursive Polynomial Model Estimator1/1 -> Bus Selector1/1
  input Signal Low Pass Filter/1 -> Recursive Polynomial Model Estimator1/1  "input"
  Bus Creator1/1 -> Calculate DC Gain1/1(Params)
  Bus Selector1/1 -> Bus Creator1/1  "<A>"
  Bus Selector1/2 -> Bus Creator1/2  "<B>"
  Substract Current Offset so that the linearised model works/1 -> Scope/2, output Signal Low Pass Filter1/1  "output minus mean"
  Edge Detector1/1 -> Get_Current_Output_Offset/Enable
  Get_Current_Output_Offset/1(Hold when disabled) -> Substract Current Offset so that the linearised model works/2
  System_Output/1 -> Get_Current_Output_Offset/1(In1), Substract Current Offset so that the linearised model works/1
  Get_Current_delayed_Input_Offset/1(Hold when disabled) -> Substract Current Offset so that the linearised model works1/2
  Edge Detector/1 -> Get_Current_delayed_Input_Offset/Enable
  PT1_Tustin/1(PT1_Output) -> Gain_Filtered/1
  System_Input/1 -> System_Delay_Simulation/1  "real input"
  Vorsicht wenn resettet wird muss erst dieser Totzeitspeicher voll gelaufen sein bevor die Adaption starten darf Sonst kommt heir immer 0 raus und die Identifikation kann nicht rechnen/1 -> System_Delay_Simulation/3
  Dead_Time/1 -> System_Delay_Simulation/2
  Substract Current Offset so that the linearised model works1/1 -> Scope/1, input Signal Low Pass Filter/1  "imput delayed minus"
  System_Delay_Simulation/1 -> Substract Current Offset so that the linearised model works1/1, Get_Current_delayed_Input_Offset/1(In1)  "input delayed"
  Calculate DC Gain1/1(Calculated_Gain) -> PT1_Tustin/1(PT1_Input), Gain_Not_Filtered/1
  Start_Identification/1 -> Edge Detector1/1, Edge Detector/1, PT1_Tustin/5(Reset), output Signal Low Pass Filter1/2, input Signal Low Pass Filter/2, Recursive Polynomial Model Estimator1/3
  output Signal Low Pass Filter1/1 -> Recursive Polynomial Model Estimator1/2
  Constant/1 -> PT1_Tustin/4(Sample_Time)
  Constant1/1 -> PT1_Tustin/2(Gain_System)
  Time_Constant_Gain_Filter/1 -> PT1_Tustin/3(Time_Constant_System)
  Recursive Polynomial Model Estimator1/2 -> Estimation_Error/1

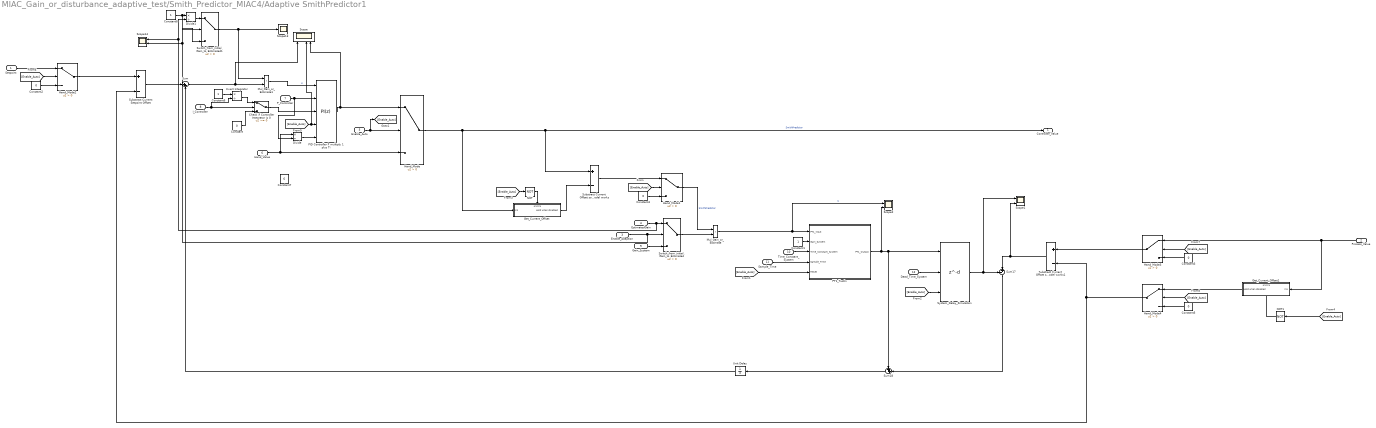
== system MIAC_Gain_or_disturbance_adaptive_test/Smith_Predictor_MIAC4/Adaptive SmithPredictor1 ==
  Setpoint : Inport
  Process_Value : Inport  Port=2
  Enable_Adaption : Inport  Port=3
  EstimatedGain : Inport  Port=4
  Enable_Auto : Inport  Port=5
  Hand_Value : Inport  Port=6
  P_Controller : Inport  Port=7
  I_Controller : Inport  Port=8
  Gain_System : Inport  Port=9
  Time_Constant_System : Inport  Port=10
  Sample_Time : Inport  Port=11
  " Dead_Time_System" : Inport  Port=12
  Check if Controller Integrator is 0 : Switch  Criteria=u2 ~= 0
  Constant{,2..5} (5 alike) : Constant  Value=0
  Constant1 : Constant
  Constant6 : Constant
  Constant7 : Constant  Value=6
  Constant8 : Constant
  Divide : Product  Inputs=*/
  Divide1 : Product  Inputs=*/
  Get_Current_Offset : Subsystem
  Get_Current_Offset1 : Subsystem
  Hand_Mode{,1..4} (5 alike) : Switch  Criteria=u2 > Threshold
  Invert Integrator : Product  Inputs=*/
  Mul_Gain_or_Estimate : Product
  Mul_Gain_or_Estimate1 : Product
  NOT : Logic  Operator=NOT  IconShape=distinctive  AllPortsSameDT=off  OutDataTypeStr=boolean
  NOT1 : Logic  Operator=NOT  IconShape=distinctive  AllPortsSameDT=off  OutDataTypeStr=boolean
  "PID Controller P multiply 1 plus Ti " : simulink/Continuous/PID Controller  Controller=PI  Form=Ideal  TimeDomain=Discrete-time  SampleTime=1  IntegratorMethod=Forward Euler  FilterMethod=Forward Euler  ControllerParametersSource=external  P=3.04732259067536  I=0.00445689106465138  D=118.272348286844  UseFilter=on  N=0.00420306193364532  TunerSelectOption=Transfer Function Based (PID Tuner App)  InitialConditionSource=external  InitialConditionForIntegrator=0  InitialConditionForFilter=0  DifferentiatorICPrevScaledInput=0  ExternalReset=rising  TrackingMode=off  Kt=1  LimitOutput=on  UpperSaturationLimit=100  LowerSaturationLimit=0  LinearizeAsGain=on  AntiWindupMode=none  Kb=1  POutMin=[]  POutMax=[]  IOutMin=[]  IOutMax=[]  DOutMin=[]  DOutMax=[]  NOutMin=[]  NOutMax=[]  SumOutMin=[]  SumOutMax=[]  SaturationOutMin=[]  SaturationOutMax=[]  PParamMin=[]  PParamMax=[]  IParamMin=[]  IParamMax=[]  DParamMin=[]  DParamMax=[]  NParamMin=[]  NParamMax=[]  KbParamMin=[]  KbParamMax=[]  KtParamMin=[]  KtParamMax=[]  KbOutMin=[]  KbOutMax=[]  KtOutMin=[]  KtOutMax=[]  IntegratorOutMin=[]  IntegratorOutMax=[]  FilterOutMin=[]  FilterOutMax=[]  SumI1OutMin=[]  SumI1OutMax=[]  SumI2OutMin=[]  SumI2OutMax=[]  SumI3OutMin=[]  SumI3OutMax=[]  SumI4OutMin=[]  SumI4OutMax=[]  SumDOutMin=[]  SumDOutMax=[]  DifferentiatorOutMin=[]  DifferentiatorOutMax=[]  FilterDiffOutCoefMin=[]  FilterDiffOutCoefMax=[]  ReciprocalOutMin=[]  ReciprocalOutMax=[]  SumDenOutMin=[]  SumDenOutMax=[]  SumNumOutMin=[]  SumNumOutMax=[]  DivideOutMin=[]  DivideOutMax=[]  IntegratorContinuousStateAttributes=''  IntegratorStateMustResolveToSignalObject=off  IntegratorRTWStateStorageClass=Auto  FilterContinuousStateAttributes=''  FilterStateMustResolveToSignalObject=off  FilterRTWStateStorageClass=Auto  ParallelPVariant=Passthrough  IdealPVariant=ExternalParameters  IVariant=ExternalParameters  DVariant=Disabled  IntegratorVariant=Discrete  SatVariant=Enabled  AWVariant=Passthrough  PCopyVariant=Disabled  TRVariant=Disabled  FdbkBlocksVariant=Forward  IdealPFdbkVariant=Disabled  SatFdbkVariant=Disabled  DerivativeFilterVariant=Disabled  NVariant=Disabled  NCopyVariant=Disabled_SignalSpec  FilterICVariant=Disabled  IntegratorICVariant=ExternalICs  ExternalResetVariant=ExternalReset  TRSumVariant=Passthrough  SumFdbkVariant=Disabled  SumVariant=Sum_PI
  PT1_Tustin : Subsystem  TreatAsAtomicUnit=on  SystemSampleTime=1
  Scope : Scope  NumInputPorts=4
  Scope1 : Scope  NumInputPorts=2
  Scope13 : Scope
  Scope14 : Scope  NumInputPorts=2
  Scope2 : Scope  NumInputPorts=2
  Substract Current Offset so that the linearised model works : Sum  Inputs=+-
  Substract Current Offset so that the linearised model works1 : Sum  Inputs=+-
  Substract Current Setpoint Offset : Sum  Inputs=+-
  Sum : Sum  Inputs=|+-
  Sum17 : Sum  Inputs=-+|
  Sum18 : Sum  Inputs=++|
  Switch_from_initial_Gain_to_Estimated : Switch  Criteria=u2 > Threshold
  Switch_from_initial_Gain_to_Estimated1 : Switch  Criteria=u2 > Threshold
  System_Delay_Simulation : Delay  DelayLengthSource=Input port  DelayLength=600  DelayLengthUpperLimit=800  ExternalReset=Rising  SampleTime=1
      settings: InputPortMap=u0,p1,r5
  Unit Delay : UnitDelay
  Controller_Value : Outport
  wires:
  Substract Current Setpoint Offset/1 -> Sum/1
  Hand_Mode/1 -> Get_Current_Offset/1(In1), Controller_Value/1, Substract Current Offset so that the linearised model works/1  "SmithPredictor"
  Substract Current Offset so that the linearised model works1/1 -> Scope1/2, Sum17/2
  PT1_Tustin/1(PT1_Output) -> Scope2/2, Sum18/1, System_Delay_Simulation/1
  System_Delay_Simulation/1 -> Scope1/1, Sum17/1
  Sum17/1 -> Sum18/2
  Mul_Gain_or_Estimate/1 -> Scope2/1, PT1_Tustin/1(PT1_Input)  "U"
  Switch_from_initial_Gain_to_Estimated/1 -> Mul_Gain_or_Estimate/2
  "PID Controller P multiply 1 plus Ti "/1 -> Hand_Mode/1, Scope/4
  Hand_Value/1 -> Divide/1, Hand_Mode/3
  Enable_Auto/1 -> [Enable_Auto], Hand_Mode/2
  P_Controller/1 -> Divide/2, "PID Controller P multiply 1 plus Ti "/2
  Check if Controller Integrator is 0/1 -> "PID Controller P multiply 1 plus Ti "/3
  " Dead_Time_System"/1 -> System_Delay_Simulation/2
  Gain_System/1 -> Switch_from_initial_Gain_to_Estimated/3
  [Enable_Auto] -> Hand_Mode1/2
  Hand_Mode1/1 -> Mul_Gain_or_Estimate/1  "SmithPredictor"
  Constant4/1 -> Hand_Mode1/3
  [Enable_Auto] -> PT1_Tustin/5(Reset)
  [Enable_Auto] -> System_Delay_Simulation/3
  Substract Current Offset so that the linearised model works/1 -> Hand_Mode1/1
  Get_Current_Offset/1(Hold when disabled) -> Substract Current Offset so that the linearised model works/2
  [Enable_Auto] -> NOT/1
  NOT/1 -> Get_Current_Offset/Enable
  Sum18/1 -> Unit Delay/1
  Hand_Mode2/1 -> Substract Current Setpoint Offset/1
  NOT1/1 -> Get_Current_Offset1/Enable
  [Enable_Auto] -> NOT1/1
  Hand_Mode4/1 -> Substract Current Setpoint Offset/2, Substract Current Offset so that the linearised model works1/2
  Setpoint/1 -> Hand_Mode2/1
  [Enable_Auto] -> Hand_Mode2/2
  Constant2/1 -> Hand_Mode2/3
  Process_Value/1 -> Get_Current_Offset1/1(In1), Hand_Mode3/1
  [Enable_Auto] -> Hand_Mode3/2
  Constant3/1 -> Hand_Mode3/3
  Hand_Mode3/1 -> Substract Current Offset so that the linearised model works1/1
  Constant5/1 -> Hand_Mode4/3
  [Enable_Auto] -> Hand_Mode4/2
  Get_Current_Offset1/1(Hold when disabled) -> Hand_Mode4/1
  Time_Constant_System/1 -> PT1_Tustin/3(Time_Constant_System)
  Constant1/1 -> PT1_Tustin/2(Gain_System)
  Sample_Time/1 -> PT1_Tustin/4(Sample_Time)
  I_Controller/1 -> Check if Controller Integrator is 0/2, Invert Integrator/2
  Constant/1 -> Check if Controller Integrator is 0/3
  Invert Integrator/1 -> Check if Controller Integrator is 0/1
  Constant6/1 -> Invert Integrator/1
  Unit Delay/1 -> Sum/2
  [Enable_Auto] -> Scope/3, "PID Controller P multiply 1 plus Ti "/4
  Divide/1 -> "PID Controller P multiply 1 plus Ti "/5
  Enable_Adaption/1 -> Switch_from_initial_Gain_to_Estimated/2, Switch_from_initial_Gain_to_Estimated1/2, Scope14/2
  Sum/1 -> Scope/1, Mul_Gain_or_Estimate1/2
  Switch_from_initial_Gain_to_Estimated1/1 -> Mul_Gain_or_Estimate1/1, Scope13/1
  Divide1/1 -> Switch_from_initial_Gain_to_Estimated1/1
  Constant8/1 -> Switch_from_initial_Gain_to_Estimated1/3, Divide1/1
  EstimatedGain/1 -> Switch_from_initial_Gain_to_Estimated/1, Scope14/1, Divide1/2
  Mul_Gain_or_Estimate1/1 -> "PID Controller P multiply 1 plus Ti "/1  "U"

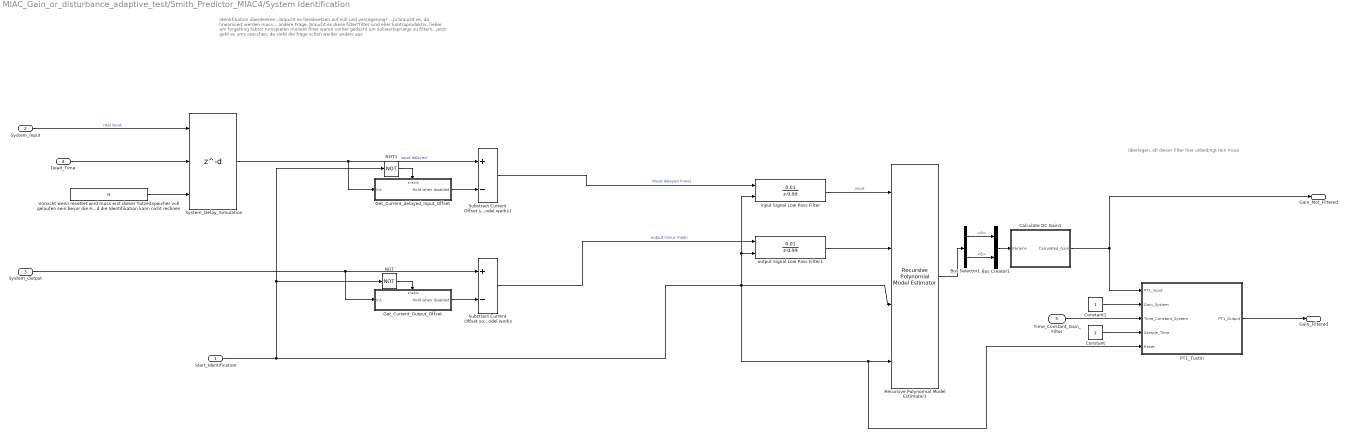
== system MIAC_Gain_or_disturbance_adaptive_test/Smith_Predictor_MIAC4/System Identification ==
  note: überlegen, ob dieser filter hier unbedingt rein muss
  note: Identifikation überdenken...braucht es herabsetzen auf null und verzögerung?
      | ...ja braucht es, da linearisiert werden muss...
      |
      | andere Frage, braucht es diese filter?filter sind eher kontraproduktiv, lieber am forgetting faktor rumspielen
      | monent fliter waren vorher gedacht um sollwertsprünge zu filtern...jetzt geht es ums rauschen, da sieht die frage schon weider anders aus
  Start_Identification : Inport  SampleTime=1
  System_Input : Inport  Port=2
  System_Output : Inport  Port=3  SampleTime=1
  Dead_Time : Inport  Port=4
  Time_Constant_Gain_Filter : Inport  Port=5
  Bus Creator1 : BusCreator  Inputs=2
  Bus Selector1 : BusSelector  OutputSignals=A,B
  Calculate DC Gain1 : Subsystem  TreatAsAtomicUnit=on  SystemSampleTime=1
  Constant : Constant
  Constant1 : Constant
  Get_Current_Output_Offset : Subsystem
  Get_Current_delayed_Input_Offset : Subsystem
  NOT : Logic  Operator=NOT  IconShape=distinctive  AllPortsSameDT=off  OutDataTypeStr=boolean
  NOT1 : Logic  Operator=NOT  IconShape=distinctive  AllPortsSameDT=off  OutDataTypeStr=boolean
  PT1_Tustin : Subsystem  TreatAsAtomicUnit=on  SystemSampleTime=1
  Recursive Polynomial Model Estimator1 : slident/Estimators/Recursive Polynomial Model Estimator  ModelStructure=ARX  InitialEstimateSource=None  A0=2  B0=1  C0=1  D0=1  F0=1  nk=1  P0=10  InitialInputs=0  InitialOutputs=0  History=Infinite  WindowLength=2000  EstimationMethod=Forgetting Factor  AdaptationParameter=1  HasTimeVaryingAdaptationParameter=off  NormalizationBias=eps  OutputError=off  OutputP=off  AddEnablePort=on  ExternalReset=Rising  InputProcessing=Sample-based  Ts=1
      settings: SourceProductName=System Identification Toolbox  SourceProductBaseCode=ID
  Substract Current Offset so that the linearised model works : Sum  Inputs=+-
  Substract Current Offset so that the linearised model works1 : Sum  Inputs=+-
  System_Delay_Simulation : Delay  DelayLengthSource=Input port  DelayLength=600  DelayLengthUpperLimit=800  ExternalReset=Rising  SampleTime=1
      settings: InputPortMap=u0,p1,r5
  Vorsicht wenn resettet wird muss erst dieser Totzeitspeicher voll gelaufen sein bevor die Adaption starten darf Sonst kommt heir immer 0 raus und die Identifikation kann nicht rechnen : Constant  Value=0
  input Signal Low Pass Filter : DiscreteTransferFcn  Numerator=[0.01]  Denominator=[1 -0.99]  ExternalReset=Rising  SampleTime=1  a0EqualsOne=on
      settings: InputPortMap=u0,r7
  output Signal Low Pass Filter1 : DiscreteTransferFcn  Numerator=[0.01]  Denominator=[1 -0.99]  ExternalReset=Rising  SampleTime=1  a0EqualsOne=on
      settings: InputPortMap=u0,r7
  Gain_Filtered : Outport
  Gain_Not_Filtered : Outport  Port=2
  wires:
  Recursive Polynomial Model Estimator1/1 -> Bus Selector1/1
  input Signal Low Pass Filter/1 -> Recursive Polynomial Model Estimator1/1  "input"
  Bus Creator1/1 -> Calculate DC Gain1/1(Params)
  Bus Selector1/1 -> Bus Creator1/1  "<A>"
  Bus Selector1/2 -> Bus Creator1/2  "<B>"
  Substract Current Offset so that the linearised model works/1 -> output Signal Low Pass Filter1/1  "output minus mean"
  NOT/1 -> Get_Current_Output_Offset/Enable
  Get_Current_Output_Offset/1(Hold when disabled) -> Substract Current Offset so that the linearised model works/2
  System_Output/1 -> Get_Current_Output_Offset/1(In1), Substract Current Offset so that the linearised model works/1
  Get_Current_delayed_Input_Offset/1(Hold when disabled) -> Substract Current Offset so that the linearised model works1/2
  NOT1/1 -> Get_Current_delayed_Input_Offset/Enable
  PT1_Tustin/1(PT1_Output) -> Gain_Filtered/1
  System_Input/1 -> System_Delay_Simulation/1  "real input"
  Vorsicht wenn resettet wird muss erst dieser Totzeitspeicher voll gelaufen sein bevor die Adaption starten darf Sonst kommt heir immer 0 raus und die Identifikation kann nicht rechnen/1 -> System_Delay_Simulation/3
  Dead_Time/1 -> System_Delay_Simulation/2
  Substract Current Offset so that the linearised model works1/1 -> input Signal Low Pass Filter/1  "imput delayed minus"
  System_Delay_Simulation/1 -> Substract Current Offset so that the linearised model works1/1, Get_Current_delayed_Input_Offset/1(In1)  "input delayed"
  Calculate DC Gain1/1(Calculated_Gain) -> PT1_Tustin/1(PT1_Input), Gain_Not_Filtered/1
  Start_Identification/1 -> NOT/1, NOT1/1, PT1_Tustin/5(Reset), Recursive Polynomial Model Estimator1/4, output Signal Low Pass Filter1/2, input Signal Low Pass Filter/2, Recursive Polynomial Model Estimator1/3
  output Signal Low Pass Filter1/1 -> Recursive Polynomial Model Estimator1/2
  Constant/1 -> PT1_Tustin/4(Sample_Time)
  Constant1/1 -> PT1_Tustin/2(Gain_System)
  Time_Constant_Gain_Filter/1 -> PT1_Tustin/3(Time_Constant_System)

== system MIAC_Gain_or_disturbance_adaptive_test/Smith_Predictor_MIAC/Adaptive SmithPredictor1/Get_Current_Offset ==
  In1 : Inport
  Enable : EnablePort
  Hold when disabled : Outport
  wires:
  In1/1 -> Hold when disabled/1

== system MIAC_Gain_or_disturbance_adaptive_test/Smith_Predictor_MIAC/Adaptive SmithPredictor1/Get_Current_Offset1 ==
  In1 : Inport
  Enable : EnablePort
  Hold when disabled : Outport
  wires:
  In1/1 -> Hold when disabled/1
